simulink model "MIMO_Drone_OpenLoopModel"  (R2025b)
settings: Solver=VariableStepAuto  StartTime=0.0  StopTime=10.0  RelTol=1e-3
undefined symbols (not defined in the file or in its folder): est_ss_n4sid
libraries: Drone_MIMO_Simple_Model x1
settings Model: Creator=Alek  LastModifiedBy=Alek

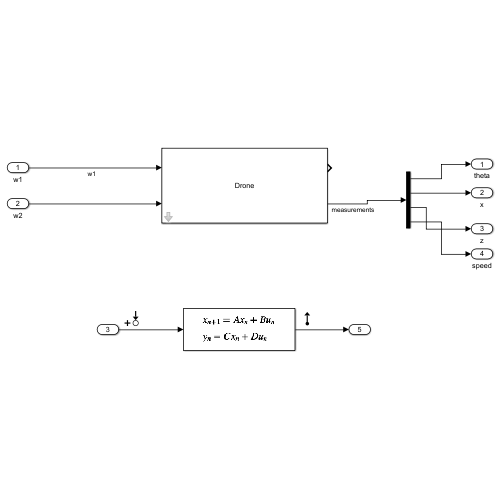
[thumbnail: Simulink's stored preview of the top-level diagram]
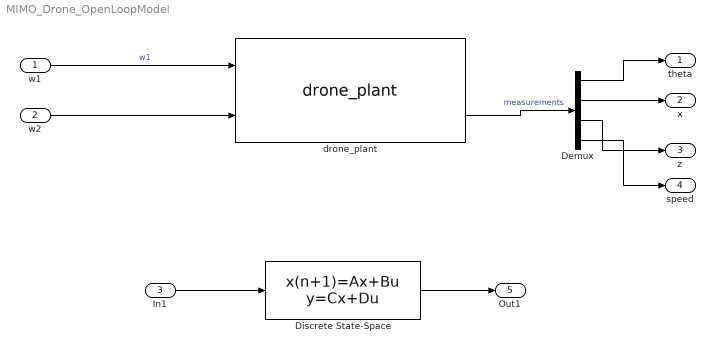
== system MIMO_Drone_OpenLoopModel ==
  w1 : Inport
  w2 : Inport  Port=2
  In1 : Inport  Port=3  PortDimensions=2
  Demux : Demux
  Discrete State-Space : DiscreteStateSpace  A=est_ss_n4sid.A  B=est_ss_n4sid.B  C=est_ss_n4sid.C  D=est_ss_n4sid.D  InitialCondition=[0 0 0 0 0 0 0 0 0 0]  SampleTime=0.00001
  drone_plant : Drone_MIMO_Simple_Model/drone_plant  kf=1e-5  m=0.5  l=1e-2  Irod=6.6666e-5
      settings: SourceProductName=DroneLibrary
  theta : Outport
  x : Outport  Port=2
  z : Outport  Port=3
  speed : Outport  Port=4
  Out1 : Outport  Port=5  PortDimensions=4
  wires:
  w1/1 -> drone_plant/1  "w1"
  w2/1 -> drone_plant/2
  drone_plant/2 -> Demux/1  "measurements"
  Demux/1 -> theta/1
  Demux/2 -> x/1
  Demux/3 -> z/1
  Demux/4 -> speed/1
  In1/1 -> Discrete State-Space/1
  Discrete State-Space/1 -> Out1/1
